simulink model "sine_fit"  (R2018a)
settings: Solver=VariableStepAuto  StartTime=0.0  StopTime=10.0  RelTol=1e-3
settings Model: Creator=berke  LastModifiedBy=berke

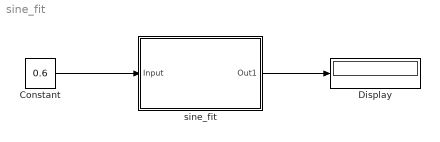
== system sine_fit ==
  Constant : Constant  Value=0.6  OutDataTypeStr=fixdt(1,8,7)  SampleTime=0.1
  Display : Display
  sine_fit : Subsystem
  wires:
  Constant/1 -> sine_fit/1(Input)
  sine_fit/1(Out1) -> Display/1

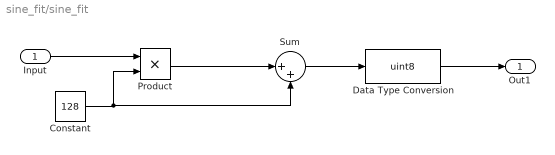
== system sine_fit/sine_fit ==
  Input : Inport  OutDataTypeStr=fixdt(1,8,7)  SampleTime=0.1
  Constant : Constant  Value=128  OutDataTypeStr=fixdt(0,8,0)  SampleTime=0.1
  Data Type Conversion : DataTypeConversion  OutDataTypeStr=uint8
  Product : Product
  Sum : Sum  Inputs=|++
  Out1 : Outport
  wires:
  Constant/1 -> Sum/2, Product/2
  Input/1 -> Product/1
  Product/1 -> Sum/1
  Sum/1 -> Data Type Conversion/1
  Data Type Conversion/1 -> Out1/1
